simulink model "lab2_EmulationSS_ContinuosTime_Robust_IntegralAction"  (R2020b)
settings: Solver=VariableStepAuto  StartTime=0.0  StopTime=10.0  RelTol=1e-3
undefined symbols (not defined in the file): A0, B0, C0, D0, Ke, Nu, Nx, sens, stepAmplitude
settings Model: Creator=Musta  LastModifiedBy=Musta

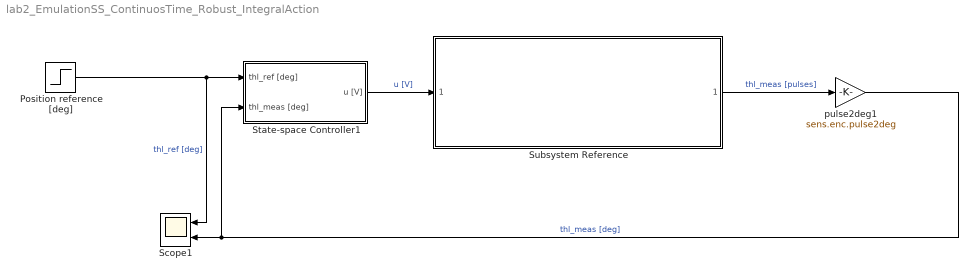
== system lab2_EmulationSS_ContinuosTime_Robust_IntegralAction ==
  Position reference [deg] : Step  Time=0  After=stepAmplitude  SampleTime=0
  Scope1 : Scope  NumInputPorts=2
  State-space Controller1 : Subsystem
  Subsystem Reference : Subsystem  ReferencedSubsystem=plant_model
  pulse2deg1 : Gain  Gain=sens.enc.pulse2deg
  wires:
  pulse2deg1/1 -> State-space Controller1/2(thl_meas [deg]), Scope1/2  "thl_meas [deg]"
  Position reference [deg]/1 -> Scope1/1, State-space Controller1/1(thl_ref [deg])  "thl_ref [deg]"
  Subsystem Reference/1 -> pulse2deg1/1  "thl_meas [pulses]"
  State-space Controller1/1(u [V]) -> Subsystem Reference/1  "u [V]"

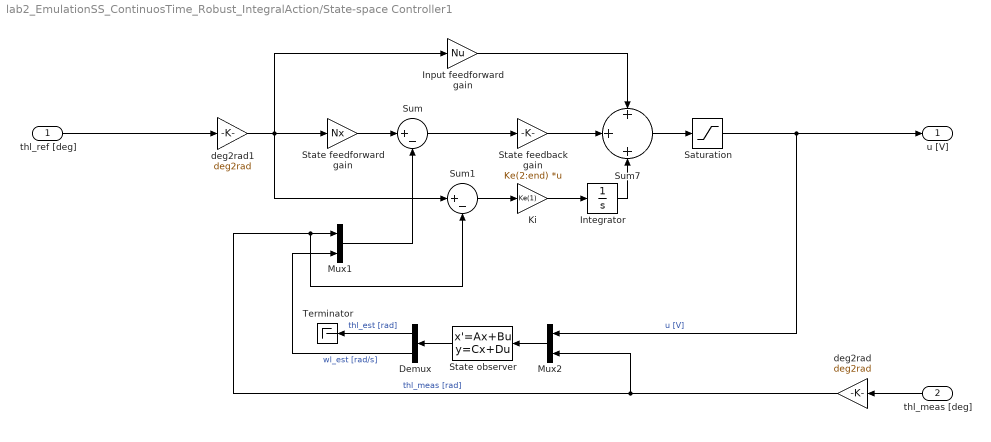
== system lab2_EmulationSS_ContinuosTime_Robust_IntegralAction/State-space Controller1 ==
  thl_ref [deg] : Inport
  thl_meas [deg] : Inport  Port=2
  Demux : Demux  Outputs=2
  Input feedforward gain : Gain  Gain=Nu
  Integrator : Integrator
  Ki : Gain  Gain=Ke(1)
  Mux1 : Mux  Inputs=2
  Mux2 : Mux  Inputs=2
  Saturation : Saturate  UpperLimit=10  LowerLimit=-10
  "State feedback gain " : Gain  Gain=Ke(2:end)  Multiplication=Matrix(K*u)
  State feedforward gain : Gain  Gain=Nx
  State observer : StateSpace  A=A0  B=B0  C=C0  D=D0  InitialCondition=0
  Sum : Sum  Inputs=|+-
  Sum1 : Sum  Inputs=|+-
  Sum7 : Sum  Inputs=+||+||+
  Terminator : Terminator
  deg2rad : Gain  Gain=deg2rad
  deg2rad1 : Gain  Gain=deg2rad
  u [V] : Outport
  wires:
  "State feedback gain "/1 -> Sum7/2
  Sum1/1 -> Ki/1
  thl_meas [deg]/1 -> deg2rad/1
  Integrator/1 -> Sum7/3
  Input feedforward gain/1 -> Sum7/1
  Ki/1 -> Integrator/1
  Sum/1 -> "State feedback gain "/1
  Mux1/1 -> Sum/2
  Sum7/1 -> Saturation/1
  deg2rad1/1 -> Sum1/1, Input feedforward gain/1, State feedforward gain/1
  thl_ref [deg]/1 -> deg2rad1/1
  State feedforward gain/1 -> Sum/1
  Demux/1 -> Terminator/1  "thl_est [rad]"
  Saturation/1 -> Mux2/1, u [V]/1  "u [V]"
  State observer/1 -> Demux/1
  Mux2/1 -> State observer/1
  Demux/2 -> Mux1/2  "wl_est [rad/s]"
  deg2rad/1 -> Sum1/2, Mux1/1, Mux2/2  "thl_meas [rad]"
